simulink model "result"  (R2016b)
settings: Solver=VariableStepAuto  StartTime=0.0  StopTime=10.0  RelTol=1e-3
settings Model: Creator=Hasee  LastModifiedBy=Hasee

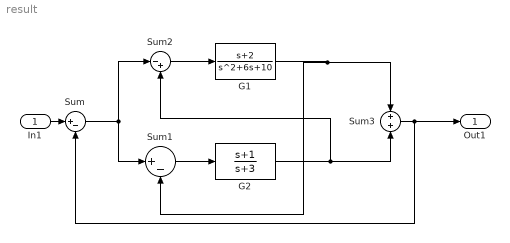
== system result ==
  In1 : Inport
  G1 : TransferFcn  Numerator=[1,2]  Denominator=[1,6,10]
  "G2 " : TransferFcn  Numerator=[1,1]  Denominator=[1,3]
  Sum : Sum  Inputs=|+-
  Sum1 : Sum  Inputs=|+-
  Sum2 : Sum  Inputs=|-+
  Sum3 : Sum
  Out1 : Outport
  wires:
  Sum2/1 -> G1/1
  Sum/1 -> Sum2/1, Sum1/1
  "G2 "/1 -> Sum2/2, Sum3/2
  G1/1 -> Sum1/2, Sum3/1
  Sum1/1 -> "G2 "/1
  Sum3/1 -> Out1/1, Sum/2
  In1/1 -> Sum/1
